simulink model "vehicule_all_controller_step"  (R2024a)
settings: Solver=VariableStepAuto  StartTime=0.0  StopTime=4.5  RelTol=1e-3
libraries: fuzblock x2, slpidlib x2, simulink x1
settings Model: Creator=idial068  LastModifiedBy=odaal085

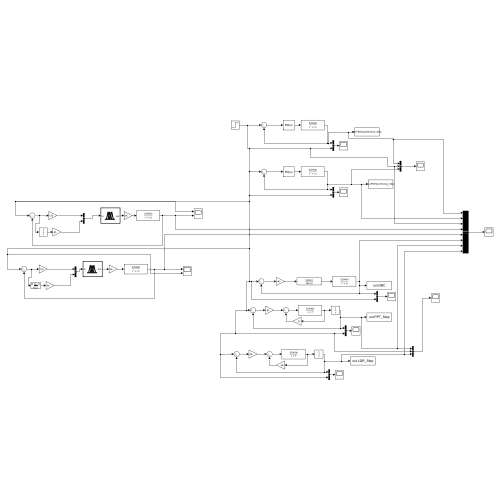
[thumbnail: Simulink's stored preview of the top-level diagram]
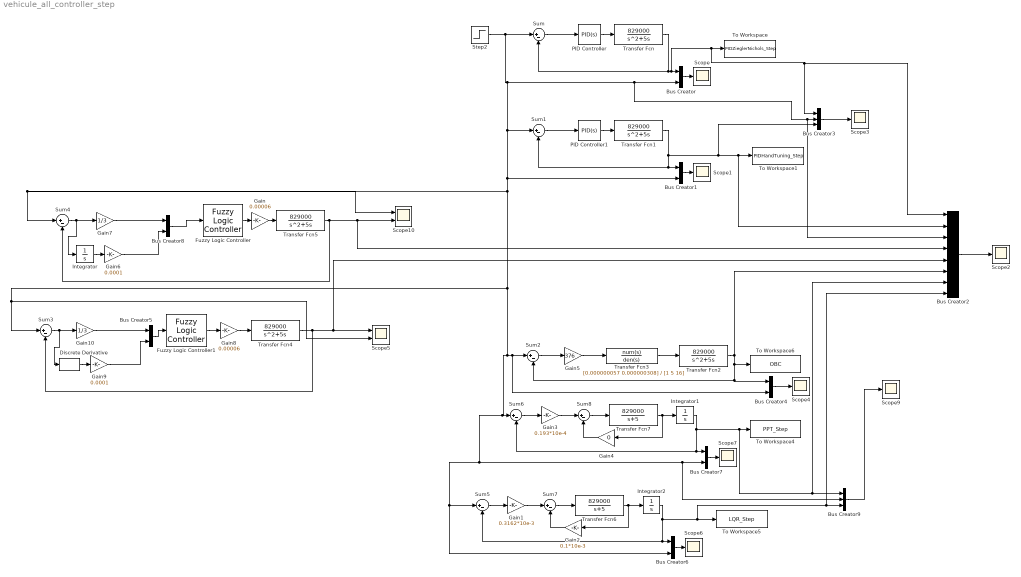
== system vehicule_all_controller_step ==
  Bus Creator{,1,4..8} (7 alike) : BusCreator  Inputs=2
  Bus Creator2 : BusCreator  Inputs=8
  Bus Creator3 : BusCreator  Inputs=3
  Bus Creator9 : BusCreator  Inputs=3
  Discrete Derivative : simulink/Discrete/Discrete Derivative  gainval=1.0  ICPrevScaledInput=0.0  OutMin=[]  OutMax=[]  OutDataType=fixdt(1, 16)  OutScaling=2^-10  DoSatur=off
  Fuzzy Logic Controller : fuzblock/Fuzzy Logic  Controller  FIS='FLC.fis'  OutputSampleNumber=101  DataType=double  FuzzifiedInputs=off  RuleFiringStrengths=off  RuleOutputs=off  AggregatedOutputs=off  SimulateUsing=Interpreted execution  OutOfRangeInputValueMessage=warning  NoRuleFiredMessage=warning  EmptyOutputFuzzySetMessage=warning
  Fuzzy Logic Controller1 : fuzblock/Fuzzy Logic  Controller  FIS='FLC.fis'  OutputSampleNumber=101  DataType=double  FuzzifiedInputs=off  RuleFiringStrengths=off  RuleOutputs=off  AggregatedOutputs=off  SimulateUsing=Interpreted execution  OutOfRangeInputValueMessage=warning  NoRuleFiredMessage=warning  EmptyOutputFuzzySetMessage=warning
  Gain : Gain  Gain=0.00006
  Gain1 : Gain  Gain=0.3162*10e-3
  Gain10 : Gain  Gain=1/3
  Gain2 : Gain  Gain=0.1*10e-3
  Gain3 : Gain  Gain=0.193*10e-4
  Gain4 : Gain  Gain=0
  Gain5 : Gain  Gain=376
  Gain6 : Gain  Gain=0.0001
  Gain7 : Gain  Gain=1/3
  Gain8 : Gain  Gain=0.00006
  Gain9 : Gain  Gain=0.0001
  Integrator : Integrator
  Integrator1 : Integrator
  Integrator2 : Integrator
  PID Controller : slpidlib/PID Controller  Controller=PID  Form=Parallel  TimeDomain=Continuous-time  UseExternalTs=off  SampleTime=-1  IntegratorMethod=Forward Euler  FilterMethod=Forward Euler  ControllerParametersSource=internal  P=0.00012  I=0.00047  UseKiTs=off  D=0.000068  UseExternalDerivativeSource=off  N=100  UseFilter=on  TunerSelectOption=Transfer Function Based (PID Tuner App)  InitialConditionSource=internal  InitialConditionForIntegrator=0  InitialConditionForFilter=0  DifferentiatorICPrevScaledInput=0  ExternalReset=none  TrackingMode=off  Kt=1  LimitOutput=off  SatLimitsSource=internal  UpperSaturationLimit=inf  LowerSaturationLimit=-inf  LinearizeAsGain=on  AntiWindupMode=none  Kb=1  LimitIntegrator=off  UpperIntegratorSaturationLimit=inf  LowerIntegratorSaturationLimit=-inf  POutMin=[]  POutMax=[]  IOutMin=[]  IOutMax=[]  DOutMin=[]  DOutMax=[]  NOutMin=[]  NOutMax=[]  SumOutMin=[]  SumOutMax=[]  SaturationOutMin=[]  SaturationOutMax=[]  PParamMin=[]  PParamMax=[]  IParamMin=[]  IParamMax=[]  DParamMin=[]  DParamMax=[]  NParamMin=[]  NParamMax=[]  KbParamMin=[]  KbParamMax=[]  KtParamMin=[]  KtParamMax=[]  KbOutMin=[]  KbOutMax=[]  KtOutMin=[]  KtOutMax=[]  IntegratorOutMin=[]  IntegratorOutMax=[]  FilterOutMin=[]  FilterOutMax=[]  SumI1OutMin=[]  SumI1OutMax=[]  SumI2OutMin=[]  SumI2OutMax=[]  SumI3OutMin=[]  SumI3OutMax=[]  SumI4OutMin=[]  SumI4OutMax=[]  SumDOutMin=[]  SumDOutMax=[]  DifferentiatorOutMin=[]  DifferentiatorOutMax=[]  FilterDiffOutCoefMin=[]  FilterDiffOutCoefMax=[]  ReciprocalOutMin=[]  ReciprocalOutMax=[]  SumDenOutMin=[]  SumDenOutMax=[]  SumNumOutMin=[]  SumNumOutMax=[]  DivideOutMin=[]  DivideOutMax=[]  UdiffTsProdOutMin=[]  UdiffTsProdOutMax=[]  NTsProdOutMin=[]  NTsProdOutMax=[]  UintegralTsProdOutMin=[]  UintegralTsProdOutMax=[]  UngainTsProdOutMin=[]  UngainTsProdOutMax=[]  ClampingZeroOutDataTypeStr=Inherit: Inherit via back propagation  ClampingZeroOutMin=[]  ClampingZeroOutMax=[]  FilterDenConstantOutDataTypeStr=Inherit: Inherit via back propagation  FilterDenConstantOutMin=[]  FilterDenConstantOutMax=[]  PCopyOutDataTypeStr=Inherit: Inherit via back propagation  PCopyOutMin=[]  PCopyOutMax=[]  NCopyOutDataTypeStr=Inherit: Inherit via back propagation  NCopyOutMin=[]  NCopyOutMax=[]  IntegratorContinuousStateAttributes=''  IntegratorStateMustResolveToSignalObject=off  IntegratorRTWStateStorageClass=Auto  FilterContinuousStateAttributes=''  FilterStateMustResolveToSignalObject=off  FilterRTWStateStorageClass=Auto  ParallelPVariant=InternalParameters  IdealPVariant=Disabled  IVariant=InternalParameters  DVariant=InternalParameters  IntegratorVariant=Continuous  SatVariant=Disabled  AWVariant=Passthrough  PCopyVariant=Disabled  TRVariant=Disabled  FdbkBlocksVariant=Forward  IdealPFdbkVariant=Disabled  SatFdbkVariant=Disabled  DerivativeFilterVariant=ContFilter  NVariant=InternalParameters  NCopyVariant=Disabled  FilterICVariant=InternalICsFilter  IntegratorICVariant=InternalICs  ExternalResetVariant=Disabled  TRSumVariant=Passthrough  SumFdbkVariant=Disabled  SumVariant=Sum_PID  TsampFilterVariant=InternalTs  TsampNgainVariant=Passthrough  TsampIntegralVariant=Disabled_SignalSpec  ExternalSaturationOutDataTypeStr=Inherit: Same as second input  DerivativeSourceVariant=ErrorSignal
  PID Controller1 : slpidlib/PID Controller  Controller=PID  Form=Parallel  TimeDomain=Continuous-time  UseExternalTs=off  SampleTime=-1  IntegratorMethod=Forward Euler  FilterMethod=Forward Euler  ControllerParametersSource=internal  P=0.01  I=0.03  UseKiTs=off  D=0.001  UseExternalDerivativeSource=off  N=100  UseFilter=on  TunerSelectOption=Transfer Function Based (PID Tuner App)  InitialConditionSource=internal  InitialConditionForIntegrator=0  InitialConditionForFilter=0  DifferentiatorICPrevScaledInput=0  ExternalReset=none  TrackingMode=off  Kt=1  LimitOutput=off  SatLimitsSource=internal  UpperSaturationLimit=inf  LowerSaturationLimit=-inf  LinearizeAsGain=on  AntiWindupMode=none  Kb=1  LimitIntegrator=off  UpperIntegratorSaturationLimit=inf  LowerIntegratorSaturationLimit=-inf  POutMin=[]  POutMax=[]  IOutMin=[]  IOutMax=[]  DOutMin=[]  DOutMax=[]  NOutMin=[]  NOutMax=[]  SumOutMin=[]  SumOutMax=[]  SaturationOutMin=[]  SaturationOutMax=[]  PParamMin=[]  PParamMax=[]  IParamMin=[]  IParamMax=[]  DParamMin=[]  DParamMax=[]  NParamMin=[]  NParamMax=[]  KbParamMin=[]  KbParamMax=[]  KtParamMin=[]  KtParamMax=[]  KbOutMin=[]  KbOutMax=[]  KtOutMin=[]  KtOutMax=[]  IntegratorOutMin=[]  IntegratorOutMax=[]  FilterOutMin=[]  FilterOutMax=[]  SumI1OutMin=[]  SumI1OutMax=[]  SumI2OutMin=[]  SumI2OutMax=[]  SumI3OutMin=[]  SumI3OutMax=[]  SumI4OutMin=[]  SumI4OutMax=[]  SumDOutMin=[]  SumDOutMax=[]  DifferentiatorOutMin=[]  DifferentiatorOutMax=[]  FilterDiffOutCoefMin=[]  FilterDiffOutCoefMax=[]  ReciprocalOutMin=[]  ReciprocalOutMax=[]  SumDenOutMin=[]  SumDenOutMax=[]  SumNumOutMin=[]  SumNumOutMax=[]  DivideOutMin=[]  DivideOutMax=[]  UdiffTsProdOutMin=[]  UdiffTsProdOutMax=[]  NTsProdOutMin=[]  NTsProdOutMax=[]  UintegralTsProdOutMin=[]  UintegralTsProdOutMax=[]  UngainTsProdOutMin=[]  UngainTsProdOutMax=[]  ClampingZeroOutDataTypeStr=Inherit: Inherit via back propagation  ClampingZeroOutMin=[]  ClampingZeroOutMax=[]  FilterDenConstantOutDataTypeStr=Inherit: Inherit via back propagation  FilterDenConstantOutMin=[]  FilterDenConstantOutMax=[]  PCopyOutDataTypeStr=Inherit: Inherit via back propagation  PCopyOutMin=[]  PCopyOutMax=[]  NCopyOutDataTypeStr=Inherit: Inherit via back propagation  NCopyOutMin=[]  NCopyOutMax=[]  IntegratorContinuousStateAttributes=''  IntegratorStateMustResolveToSignalObject=off  IntegratorRTWStateStorageClass=Auto  FilterContinuousStateAttributes=''  FilterStateMustResolveToSignalObject=off  FilterRTWStateStorageClass=Auto  ParallelPVariant=InternalParameters  IdealPVariant=Disabled  IVariant=InternalParameters  DVariant=InternalParameters  IntegratorVariant=Continuous  SatVariant=Disabled  AWVariant=Passthrough  PCopyVariant=Disabled  TRVariant=Disabled  FdbkBlocksVariant=Forward  IdealPFdbkVariant=Disabled  SatFdbkVariant=Disabled  DerivativeFilterVariant=ContFilter  NVariant=InternalParameters  NCopyVariant=Disabled  FilterICVariant=InternalICsFilter  IntegratorICVariant=InternalICs  ExternalResetVariant=Disabled  TRSumVariant=Passthrough  SumFdbkVariant=Disabled  SumVariant=Sum_PID  TsampFilterVariant=InternalTs  TsampNgainVariant=Passthrough  TsampIntegralVariant=Disabled_SignalSpec  ExternalSaturationOutDataTypeStr=Inherit: Same as second input  DerivativeSourceVariant=ErrorSignal
  Scope{,1..4,6..7,9} (8 alike) : Scope
  Scope10 : Scope  NumInputPorts=2
  Scope5 : Scope  NumInputPorts=2
  Step2 : Step  Time=0  SampleTime=0
  Sum{,1..8} (9 alike) : Sum  Inputs=|+-
  To Workspace : ToWorkspace  VariableName=PIDZieglerNichols_Step  SaveFormat=Timeseries  SampleTime=-1
  To Workspace1 : ToWorkspace  VariableName=PIDHandTuning_Step  SaveFormat=Timeseries  SampleTime=-1
  To Workspace4 : ToWorkspace  VariableName=PPT_Step  SaveFormat=Timeseries  SampleTime=-1
  To Workspace5 : ToWorkspace  VariableName=LQR_Step  SaveFormat=Timeseries  SampleTime=-1
  To Workspace6 : ToWorkspace  VariableName=OBC  SaveFormat=Timeseries  SampleTime=-1
  Transfer Fcn{,1..2,4..5} (5 alike) : TransferFcn  Numerator=[829000]  Denominator=[1 5 0]
  Transfer Fcn3 : TransferFcn  Numerator=[0.000000057 0.000000308]  Denominator=[1 5 16]
  Transfer Fcn6 : TransferFcn  Numerator=[829000]  Denominator=[0 1 5]
  Transfer Fcn7 : TransferFcn  Numerator=[829000]  Denominator=[0 1 5]
  wires:
  Sum8/1 -> Transfer Fcn7/1
  Gain4/1 -> Sum8/2
  Integrator1/1 -> Sum6/2, Bus Creator7/1, Bus Creator2/7, Bus Creator9/1, To Workspace4/1
  Gain3/1 -> Sum8/1
  Bus Creator9/1 -> Scope9/1
  Sum6/1 -> Gain3/1
  Bus Creator7/1 -> Scope7/1
  Integrator2/1 -> Sum5/2, Bus Creator6/1, Bus Creator2/8, Bus Creator9/3, To Workspace5/1
  Transfer Fcn6/1 -> Gain2/1, Integrator2/1
  Bus Creator6/1 -> Scope6/1
  Sum7/1 -> Transfer Fcn6/1
  Gain1/1 -> Sum7/1
  Sum1/1 -> PID Controller1/1
  Bus Creator3/1 -> Scope3/1
  Transfer Fcn/1 -> Sum/2, Bus Creator2/1, Bus Creator3/1, To Workspace/1, Bus Creator/1
  PID Controller1/1 -> Transfer Fcn1/1
  Bus Creator/1 -> Scope/1
  Bus Creator1/1 -> Scope1/1
  Sum/1 -> PID Controller/1
  Sum5/1 -> Gain1/1
  Gain2/1 -> Sum7/2
  PID Controller/1 -> Transfer Fcn/1
  Transfer Fcn7/1 -> Gain4/1, Integrator1/1
  Bus Creator2/1 -> Scope2/1
  Transfer Fcn1/1 -> Bus Creator3/3, Bus Creator2/2, To Workspace1/1, Sum1/2, Bus Creator1/1
  Gain5/1 -> Transfer Fcn3/1
  Sum2/1 -> Gain5/1
  Bus Creator4/1 -> Scope4/1
  Transfer Fcn2/1 -> Bus Creator2/6, To Workspace6/1, Bus Creator4/1, Sum2/2
  Transfer Fcn3/1 -> Transfer Fcn2/1
  Discrete Derivative/1 -> Gain9/1
  Bus Creator8/1 -> Fuzzy Logic Controller/1
  Gain6/1 -> Bus Creator8/2
  Bus Creator5/1 -> Fuzzy Logic Controller1/1
  Step2/1 -> Bus Creator1/2, Sum4/1, Scope10/1, Bus Creator6/2, Sum5/1, Bus Creator9/2, Bus Creator7/2, Sum6/1, Bus Creator4/2, Sum2/1, Sum3/1, Scope5/2, Sum1/1, Bus Creator2/3, Bus Creator3/2, Bus Creator/2, Sum/1
  Sum4/1 -> Integrator/1, Gain7/1
  Gain9/1 -> Bus Creator5/2
  Gain8/1 -> Transfer Fcn4/1
  Fuzzy Logic Controller1/1 -> Gain8/1
  Gain10/1 -> Bus Creator5/1
  Transfer Fcn5/1 -> Bus Creator2/4, Scope10/2, Sum4/2
  Gain7/1 -> Bus Creator8/1
  Sum3/1 -> Discrete Derivative/1, Gain10/1
  Fuzzy Logic Controller/1 -> Gain/1
  Gain/1 -> Transfer Fcn5/1
  Transfer Fcn4/1 -> Bus Creator2/5, Scope5/1, Sum3/2
  Integrator/1 -> Gain6/1
